simulink model "DR_DigitalTwin_Day2"  (R2026a)
settings: Solver=VariableStepAuto  StopTime=28512000
StartFcn:
  | queueWaitStats([], true);
undefined symbols (not defined in the file): m, n
settings Model: Creator=dell  LastModifiedBy=dell

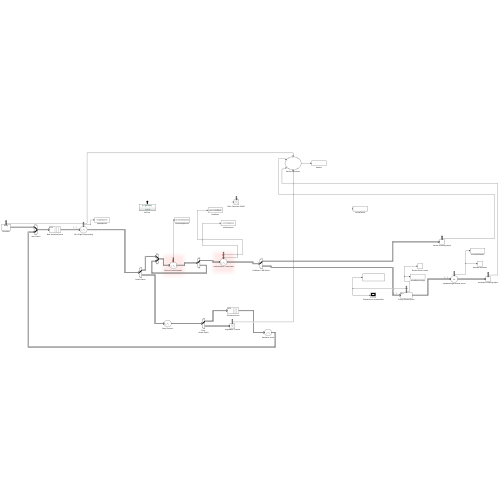
[thumbnail: Simulink's stored preview of the top-level diagram]
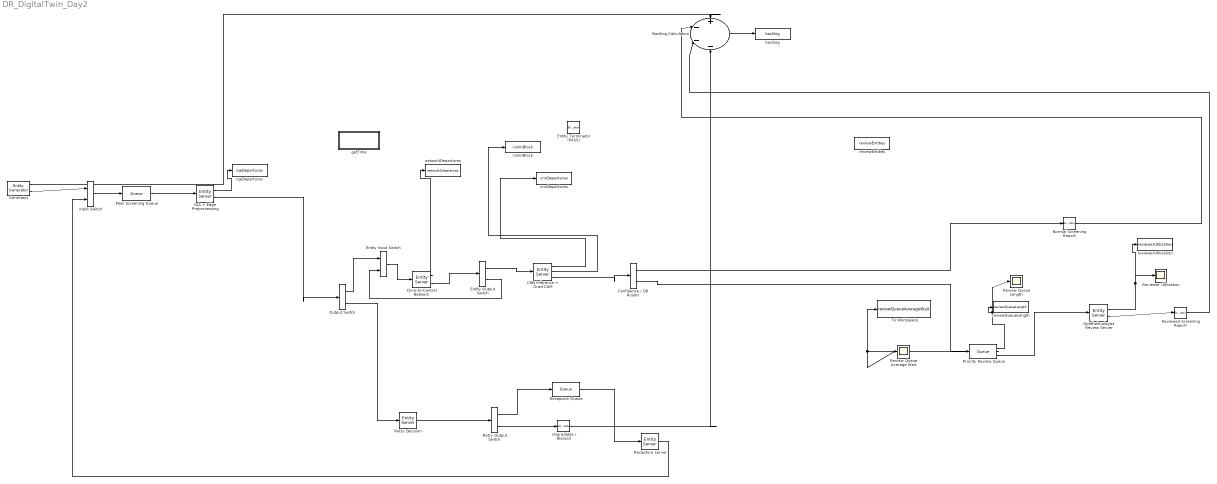
== system DR_DigitalTwin_Day2 ==
  Backlog Calculation : Sum  Inputs=+---
  CNN Inference + Grad-CAM : EntityServer  InputPortMessageModes=m  OutputPortMessageModes=n,n,m  Capacity=1  ServiceTimeValue=simParams.ai.processingTime  ServiceCompleteAction=|  NumberEntitiesDeparted=on  NumberEntitiesInBlock=on
      | if manualReviewEnabled
      | 
      |     entity.review_route = 2;
      | 
      | else
      | 
      |     if entity.confidence_level == 3 || entity.dr_severity >= 2
      |         entity.review_route = 2;
      |     else
      |         entity.review_route = 1;
      |     end
      | 
      | end
      settings: OutputPortMap=o0,o1,o9
  Clinic-to-Central Network : EntityServer  InputPortMessageModes=m  OutputPortMessageModes=n,m  Capacity=1  ServiceTimeValue=simParams.network.delay  ServiceCompleteAction=|  NumberEntitiesDeparted=on
      | if networkDropoutEnabled && rand() < networkDropoutProbability
      |     entity.network_route = 2;
      | else
      |     entity.network_route = 1;
      | end
      settings: OutputPortMap=o0,o9
  Confidence / DR Router : EntityOutputSwitch  InputPortMessageModes=m  OutputPortMessageModes=m,m  SwitchingCriterion=From attribute  SwitchAttributeName=review_route
  Entity Input Switch : EntityInputSwitch  InputPortMessageModes=m,m  OutputPortMessageModes=m
  Entity Output Switch : EntityOutputSwitch  InputPortMessageModes=m  OutputPortMessageModes=m,m  SwitchingCriterion=From attribute  SwitchAttributeName=network_route
  Entity Terminator (PASS) : EntityTerminator  InputPortMessageModes=m  NumberEntitiesArrived=on
      settings: OutputPortMap=o0
  Generator : EntityGenerator  OutputPortMessageModes=n,m  TimeSource=MATLAB action  IntergenerationTimeAction=dt = -(1/arrivalRate)*log(1-rand());  AttributeName=retry_count|iqa_status|dr_severity|confidence_level|iqa_route|retry_route|review_route|review_priority|review_time|queue_entry_time|queue_wait_time|network_route  AttributeInitialValue=0|0|2|3|1|1|1|1| reviewProcessingTime|0|0|1  NumberEntitiesDeparted=on  EntityType=Structured  EntityTypeName=Entity
      settings: OutputPortMap=o0,o3
  IQA + Edge Preprocessing : EntityServer  InputPortMessageModes=m  OutputPortMessageModes=n,m  Capacity=1  ServiceTimeValue=2  EntryAction=entity.iqa_status = double(rand >= iqaFailRate);  ServiceCompleteAction=|  NumberEntitiesDeparted=on
      | if entity.iqa_status == 0
      | 
      |     if entity.retry_count < maxRetries
      |         entity.retry_count = entity.retry_count + 1;
      |         entity.retry_route = 1;
      |     else
      |         entity.retry_route = 2;
      |     end
      | 
      | else
      | 
      |     entity.retry_route = 2;
      | 
      | end
      | 
      | entity.iqa_route = entity.iqa_status + 1;
      settings: OutputPortMap=o0,o9
  Input Switch : EntityInputSwitch  InputPortMessageModes=m,m  OutputPortMessageModes=m
  Main Screening Queue : Queue  InputPortMessageModes=m  OutputPortMessageModes=m
  Normal Screening Report : EntityTerminator  InputPortMessageModes=m  NumberEntitiesArrived=on
      settings: OutputPortMap=o0
  Ophthalmologist Review Server : EntityServer  InputPortMessageModes=m  OutputPortMessageModes=n,m  Capacity=simParams.review.reviewerCount  ServiceTimeSource=Attribute  ServiceTimeValue=simParams.review.manualTime  ServiceTimeAttributeName=review_time  EntryAction=|  Utilization=on
      | entity.queue_wait_time = getTime() - entity.queue_entry_time;
      | queueWaitStats(entity.queue_wait_time, false);
      settings: OutputPortMap=o5,o9
  Output Switch : EntityOutputSwitch  InputPortMessageModes=m  OutputPortMessageModes=m,m  SwitchingCriterion=From attribute  SwitchAttributeName=iqa_route
  Priority Review Queue : Queue  InputPortMessageModes=m  OutputPortMessageModes=n,n,m  QueueType=Priority  PrioritySource=confidence_level  SortingDirection=Descending  EntryAction=entity.queue_entry_time = getTime();  NumberEntitiesInBlock=on  AverageWait=on
      settings: OutputPortMap=o1,o2,o5
  Recapture Queue : Queue  InputPortMessageModes=m  OutputPortMessageModes=m
  Recapture server : EntityServer  InputPortMessageModes=m  OutputPortMessageModes=m  Capacity=1  ServiceCompleteAction=entity.retry_count = entity.retry_count + 1;
  Retry Output Switch : EntityOutputSwitch  InputPortMessageModes=m  OutputPortMessageModes=m,m  SwitchingCriterion=From attribute  SwitchAttributeName=retry_route
  Retry Decision : EntityServer  InputPortMessageModes=m  OutputPortMessageModes=m  Capacity=1  ServiceCompleteAction=|
      | if entity.retry_count < maxRetries
      |     entity.retry_route = 1;
      | else
      |     entity.retry_route = 2;
      | end
  Review Queue Average Wait : Scope
  Review Queue Length : Scope
      settings: DataLoggingVariableName=ScopeData2
  Reviewed Screening Report : EntityTerminator  InputPortMessageModes=m  NumberEntitiesArrived=on
      settings: OutputPortMap=o0
  Reviewer Utilization : Scope
  To Workspace : ToWorkspace  VariableName=reviewQueueAverageWait  SaveFormat=Timeseries  SampleTime=-1
  Ungradable / Discard : EntityTerminator  InputPortMessageModes=m  NumberEntitiesArrived=on
      settings: OutputPortMap=o0
  backlog : ToWorkspace  VariableName=backlog  SaveFormat=Timeseries  SampleTime=-1
  cnnDepartures : ToWorkspace  VariableName=cnnDepartures  SaveFormat=Timeseries  SampleTime=-1
  cnnInBlock : ToWorkspace  VariableName=cnnInBlock  SaveFormat=Timeseries  SampleTime=-1
  getTime : Subsystem  TreatAsAtomicUnit=on
  iqaDepartures : ToWorkspace  VariableName=iqaDepartures  SaveFormat=Timeseries  SampleTime=-1
  networkDepartures : ToWorkspace  VariableName=networkDepartures  SaveFormat=Timeseries  SampleTime=-1
  reviewEntities : ToWorkspace  VariableName=reviewEntities  SaveFormat=Timeseries  SampleTime=-1
  reviewQueueLength : ToWorkspace  VariableName=reviewQueueLength  SaveFormat=Timeseries  SampleTime=-1
  reviewerUtilization : ToWorkspace  VariableName=reviewerUtilization  SaveFormat=Timeseries  SampleTime=-1
  wires:
  Input Switch/1 -> Main Screening Queue/1
  Recapture Queue/1 -> Recapture server/1
  Generator/2 -> Input Switch/1
  Output Switch/2 -> Retry Decision/1
  Recapture server/1 -> Input Switch/2
  IQA + Edge Preprocessing/2 -> Output Switch/1
  Retry Decision/1 -> Retry Output Switch/1
  Retry Output Switch/1 -> Recapture Queue/1
  Retry Output Switch/2 -> Ungradable / Discard/1
  Priority Review Queue/3 -> Ophthalmologist Review Server/1
  CNN Inference + Grad-CAM/3 -> Confidence / DR Router/1
  Priority Review Queue/2 -> To Workspace/1, Review Queue Average Wait/1
  Ophthalmologist Review Server/1 -> Reviewer Utilization/1, reviewerUtilization/1
  Ophthalmologist Review Server/2 -> Reviewed Screening Report/1
  Confidence / DR Router/1 -> Normal Screening Report/1
  Confidence / DR Router/2 -> Priority Review Queue/1
  Generator/1 -> Backlog Calculation/1
  Normal Screening Report/1 -> Backlog Calculation/2
  Reviewed Screening Report/1 -> Backlog Calculation/3
  Ungradable / Discard/1 -> Backlog Calculation/4
  Backlog Calculation/1 -> backlog/1
  Priority Review Queue/1 -> Review Queue Length/1, reviewQueueLength/1
  CNN Inference + Grad-CAM/1 -> cnnDepartures/1
  CNN Inference + Grad-CAM/2 -> cnnInBlock/1
  Clinic-to-Central Network/1 -> networkDepartures/1
  IQA + Edge Preprocessing/1 -> iqaDepartures/1
  Clinic-to-Central Network/2 -> Entity Output Switch/1
  Entity Output Switch/1 -> CNN Inference + Grad-CAM/1
  Entity Output Switch/2 -> Entity Input Switch/2
  Output Switch/1 -> Entity Input Switch/1
  Entity Input Switch/1 -> Clinic-to-Central Network/1
  Main Screening Queue/1 -> IQA + Edge Preprocessing/1

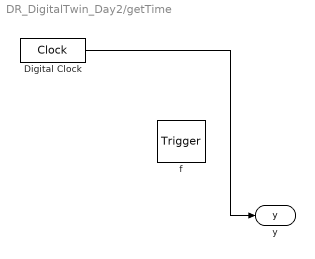
== system DR_DigitalTwin_Day2/getTime ==
  f : TriggerPort  TriggerType=function-call  IsSimulinkFunction=on  FunctionName=getTime  VariantControl=(inherit)
  Digital Clock : DigitalClock  SampleTime=-1
  y : ArgOut  DisableCoverage=on  ArgumentName=y
  wires:
  Digital Clock/1 -> y/1
